simulink library "Electric_Heater_Ctrl"  (R2018b)
settings: Solver=ode45  StartTime=0.0  StopTime=10.0  RelTol=1e-3  EnableMultiTasking=on
libraries: carnot x2
settings Model: Creator=drhf  LastModifiedBy=P41573
settings DataIOCC: LimitDataPoints=on  SaveFormat=Array  SignalLoggingSaveFormat=ModelDataLogs
settings OptimizationCC: ExpressionDepthLimit=2147483647  LifeSpan=inf
settings DebuggingCC: UnderspecifiedInitializationDetection=Classic  MergeDetectMultiDrivingBlocksExec=none  SolverPrmCheckMsg=warning  FcnCallInpInsideContextMsg=warning  StateNameClashWarn=warning  SFUnexpectedBacktrackingDiag=warning  SFNoUnconditionalDefaultTransitionDiag=warning  SFExecutionAtInitializationDiag=none
settings HardwareCC: ProdBitPerPointer=32  ProdBitPerSizeT=32  ProdBitPerPtrDiffT=32  ProdLargestAtomicFloat=None  ProdIntDivRoundTo=Undefined  ProdEndianess=Unspecified  ProdWordSize=32  ProdHWDeviceType=32-bit Generic
settings ModelReferenceCC: PropagateSignalLabelsOutOfModel=off
settings SFSimCC: SimUseLocalCustomCode=off
settings RTWCC: RTWUseLocalCustomCode=off
settings CodeAppCC: StateflowObjectComments=on
settings GRTTargetCC: TargetLangStandard=C89/C90 (ANSI)  GeneratePreprocessorConditionals=Disable all  CombineOutputUpdateFcns=off  GRTInterface=on
settings ConfigComp: CovMetricSettings=dw  CovHtmlReporting=on  CovSaveCumulativeToWorkspaceVar=on  CovSaveSingleToWorkspaceVar=on  CovExternalEMLEnable=off

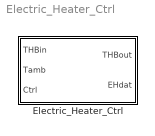
== system Electric_Heater_Ctrl ==
  Electric_Heater_Ctrl : Subsystem  mask(Electric Heater Ctrl){power=1000, UA=1, mcp=3*4182}
      mask prompts: power "Electric heating power in W"; UA "UA: thermal loss coefficient in W/K"; mcp "mcp: thermal capacity of the node in J/K"
      mask help:
      | Heats the mass flow defined in the thermo-hydraulic bus with an electric power [W]. The model has a thermal interia (Thermal Node) and losses to the ambient. The initial temperature of the thermal node is the ambient temperature.
      | mcp * dT/dt = UA*(Tamb-T) + mdot*cp_in*(Tin-T)
      |                       + Ctrl*Electric_heating_power
      | cp_in  :  heat capacity of entering fluid in J/kg/K
      | Ctrl  :  Control input, range [0...1]
      | mdot  :  entering fluid massflow in kg/s
      | Tamb : ambient temperature input in °C (for thermal losses)
      | Tin   :  temperature of entering massflow in °C
      | T     :  temperature of the node and outlet in °C
      mask Help: web(fullfile(path_carnot('help'),'Electric_Heater_Ctrl.html'),'-helpbrowser')
      mask TypeOptions power: Gain/Gain
      mask TypeOptions UA: Thermal_Node/UA
      mask TypeOptions mcp: Thermal_Node/mcp
      mask Display: plot(0,0,100,100,[50,50,60,40,50],[55,40,70,60,90],[59,50],[48,40])

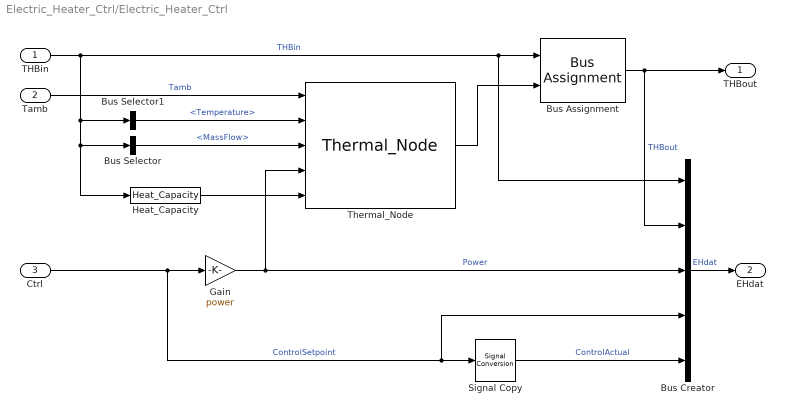
== system Electric_Heater_Ctrl/Electric_Heater_Ctrl ==
  THBin : Inport
  Tamb : Inport  Port=2
  Ctrl : Inport  Port=3
  Bus Assignment : BusAssignment  AssignedSignals=Temperature
  Bus Creator : BusCreator  Inputs=5
  Bus Selector : BusSelector  OutputSignals=MassFlow
  Bus Selector1 : BusSelector  OutputSignals=Temperature
  Gain : Gain  Gain=power
  Heat_Capacity : carnot/Basic/Material_Properties/Heat_Capacity  VariantControl=CarlibClassic  INPUTARGUMENTS=THB  DEBUGLEVEL=DEBUGLEVEL  MAXTOTALWARNINGS=inf  MAXCONSECUTIVEWARNINGS=inf  WRITETOFILE=0  FILENAME='errors.txt'
      settings: SourceProductName=Carnot
  Signal Copy : SignalConversion  OverrideOpt=off
  Thermal_Node : carnot/Basic/Thermal_Models/Thermal_Node  UA=UA  mcp=mcp
      settings: SourceProductName=Carnot
  THBout : Outport  InitialOutput=0
  EHdat : Outport  Port=2  InitialOutput=0
  wires:
  Heat_Capacity/1 -> Thermal_Node/5
  Thermal_Node/1 -> Bus Assignment/2
  Tamb/1 -> Thermal_Node/1  "Tamb"
  Signal Copy/1 -> Bus Creator/5  "ControlActual"
  Gain/1 -> Bus Creator/3, Thermal_Node/4  "Power"
  Bus Creator/1 -> EHdat/1  "EHdat"
  Bus Selector1/1 -> Thermal_Node/2  "<Temperature>"
  Bus Selector/1 -> Thermal_Node/3  "<MassFlow>"
  Bus Assignment/1 -> THBout/1, Bus Creator/2  "THBout"
  Ctrl/1 -> Gain/1, Signal Copy/1, Bus Creator/4  "ControlSetpoint"
  THBin/1 -> Bus Assignment/1, Bus Creator/1, Bus Selector1/1, Bus Selector/1, Heat_Capacity/1  "THBin"
